simulink model "PIDTrajectory"  (R2022a)
settings: Solver=FixedStepAuto  StartTime=0.0  StopTime=10.0  FixedStep=1/200  RelTol=1e-3
model workspace (MAT data in the model file):
  Fa = 200
  Kd = 600
  Kp = 90000
  M = [0 0 0 0 0 0 0 0 0 0 0 0 ... (3145728 elements, 1024x1024x3)]
  TOSEND = Simulink.NumericType
  TOSEND.DataTypeMode = 'Double'
  TOSEND.SignednessBool = 1
  TOSEND.WordLength = 64
  TOSEND.FixedExponent = 0
  TOSEND.SlopeAdjustmentFactor = 1
  TOSEND.Bias = 0
  TOSEND.DataTypeOverride = 'Inherit'
  TOSEND.IsAlias = 0
  TOSEND.DataScope = 'Auto'
  axp = [0 463.62624 872.93952 1230.15168 1537.47456 1797.12 2011.29984 2182.22592 2312.11008 2403.16416 2457.6 2477.62944 ... (510 elements, 1x510)]
  ayp = [0 -0.589653333333 -1.08202666667 -1.48224 -1.79541333333 -2.02666666667 -2.18112 -2.26389333333 -2.28010666667 -2.23488 -2.13333333333 -1.98058666667 ... (510 elements, 1x510)]
  mass = 20
  server = tcpserver.internal.TCPServer
  step = 0.01
  v0x = 0
  v0y = 0
  vxp = [0 2.3643136 9.0914816 19.6494336 33.5282176 50.24 69.3190656 90.3218176 112.8267776 136.4345856 160.768 185.4718976 ... (510 elements, 1x510)]
  vyp = [0 -0.00303146666667 -0.0114688 -0.0243648 -0.0408234666667 -0.06 -0.0811008 -0.103383466667 -0.1261568 -0.1487808 -0.170666666667 -0.1912768 ... (510 elements, 1x510)]
  x0 = 896
  xp = [896; 128]
  y0 = 895.999989756
  yp = [895.999989756; 128.007958323]
libraries: dspsrcs4 x6
(part 1 of 2)
settings Model: Creator=loryb  LastModifiedBy=loren
settings SolverCC: ShapePreserveControl=EnableAll  InsertRTBMode=Never (minimum delay)

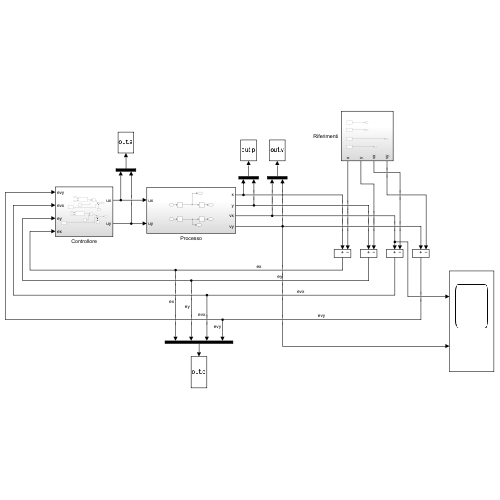
[thumbnail: Simulink's stored preview of the top-level diagram]
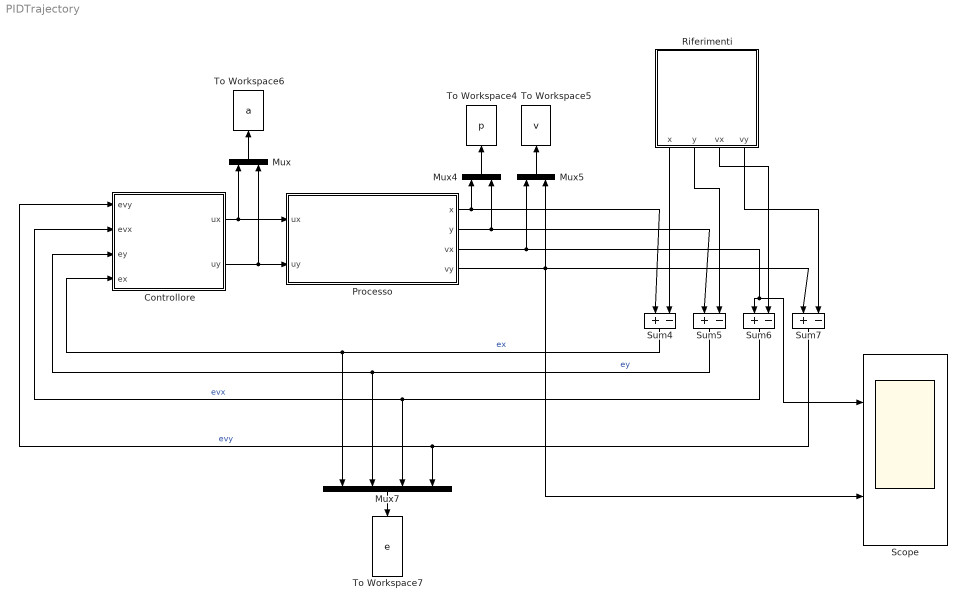
== system PIDTrajectory ==
  Controllore : Subsystem
  Mux : Mux  Inputs=2
  Mux4 : Mux  Inputs=2
  Mux5 : Mux  Inputs=2
  Mux7 : Mux
  Processo : Subsystem
  Riferimenti : Subsystem
  Scope : Scope  NumInputPorts=2
  Sum{4..7} (4 alike) : Sum  Inputs=|+-
  To Workspace4 : ToWorkspace  VariableName=p  SampleTime=-1
  To Workspace5 : ToWorkspace  VariableName=v  SampleTime=-1
      settings: Save2DSignal=2-D array (concatenate along first dimension)
  To Workspace6 : ToWorkspace  VariableName=a  SampleTime=-1
  To Workspace7 : ToWorkspace  VariableName=e  SampleTime=-1
  wires:
  Controllore/1(ux) -> Processo/1(ux), Mux/1
  Controllore/2(uy) -> Mux/2, Processo/2(uy)
  Processo/1(x) -> Mux4/1, Sum4/1
  Riferimenti/1(x) -> Sum4/2
  Processo/2(y) -> Mux4/2, Sum5/1
  Riferimenti/2(y) -> Sum5/2
  Processo/3(vx) -> Mux5/1, Scope/1, Sum6/1
  Riferimenti/3(vx) -> Sum6/2
  Processo/4(vy) -> Mux5/2, Sum7/1, Scope/2
  Riferimenti/4(vy) -> Sum7/2
  Sum4/1 -> Mux7/1, Controllore/4(ex)  "ex"
  Sum5/1 -> Controllore/3(ey), Mux7/2  "ey"
  Sum6/1 -> Mux7/3, Controllore/2(evx)  "evx"
  Sum7/1 -> Controllore/1(evy), Mux7/4  "evy"
  Mux4/1 -> To Workspace4/1
  Mux5/1 -> To Workspace5/1
  Mux7/1 -> To Workspace7/1
  Mux/1 -> To Workspace6/1
